simulink model "bh_source_WKSPACE"  (R2018a)
settings: Solver=ode4  StartTime=0.0  StopTime=80  FixedStep=0.001  RelTol=1e-5
settings Model: Creator=bhorton  LastModifiedBy=bhorton
settings SolverCC: ZeroCrossAlgorithm=Adaptive
settings OptimizationCC: LifeSpan=inf
settings DebuggingCC: SFUnexpectedBacktrackingDiag=warning  SFNoUnconditionalDefaultTransitionDiag=warning  SFExecutionAtInitializationDiag=none
settings CodeAppCC: StateflowObjectComments=on
settings GRTTargetCC: TargetLangStandard=C89/C90 (ANSI)
settings ConfigComp: CovMetricSettings=dw  CovHtmlReporting=on  CovSaveCumulativeToWorkspaceVar=on  CovSaveSingleToWorkspaceVar=on  CovExternalEMLEnable=off
settings SimscapeCC: SimscapeNormalizeSystem=off  SimscapeLogType=all  SimscapeLogDataHistory=10000  SelectedTab=Simscape Multibody
settings ExplorerConfigSet: InternalSimMechanicsExplorerSettings="<ExplorerConfiguration><canonicalview>default</canonicalview><AnimationSetting><BasePlaybackSpeed>1.0</BasePlaybackSpeed><PlaybackSpeedFactor>1.0</PlaybackSpeedFactor></AnimationSetting><TilePanel><TileInfo><Tiles Columns=\"2\" Count=\"4\" Rows=\"2\"><Column Left=\"2\" Weight=\"0.4992\"/><Column Left=\"655\" Weight=\"0.5008\"/><Column Left=\"1310\"/><Row Top=\"2\" Weight=\"0.4984\"/><Row Top=\"475\" Weight=\"0.5016\"/><Row Top=\"950\"/><Tile Height=\"1\" Width=\"1\" X=\"0\" Y=\"0\"/><Tile Height=\"1\" Width=\"1\" X=\"0\" Y=\"1\"/><Tile Height=\"1\" Width=\"1\" X=\"1\" Y=\"0\"/><Tile Height=\"1\" Width=\"1\" X=\"1\" Y=\"1\"/></Tiles></TileInfo><SceneInfo><SceneViewer><BGColor><R>0.60000002384185791</R><G>0.60000002384185791</G><B>0.60000002384185791</B></BGColor><Camera><DoPerspective>off</DoPerspective><Position><X>0.57010570867346566</X><Y>-0.81939487187068383</Y><Z>-0.041325690013103822</Z></Position><Center><X>0.57010570867346566</X><Y>0.37243777720020188</Y><Z>-0.041325690013103822</Z></Center><Up><X>0</X><Y>-0</Y><Z>1</Z></Up><ViewLimDist>1</ViewLimDist><YLim>0.58387397231837834</YLim><XLim>0.8103768064074045</XLim></Camera></SceneViewer><SceneViewer><BGColor><R>0.60000002384185791</R><G>0.60000002384185791</G><B>0.60000002384185791</B></BGColor><Camera><DoPerspective>off</DoPerspective><Position><X>0.51388092361444482</X><Y>0.52196280048326149</Y><Z>0.82022286793681332</Z></Position><Center><X>0.51388092361444482</X><Y>0.52196280048326149</Y><Z>-0.17977713206318668</Z></Center><Up><X>0</X><Y>1</Y><Z>-0</Z></Up><ViewLimDist>1</ViewLimDist><YLim>0.97737746692739225</YLim><XLim>1.3507104907751943</XLim></Camera></SceneViewer><SceneViewer><BGColor><R>0.60000002384185791</R><G>0.60000002384185791</G><B>0.60000002384185791</B></BGColor><Camera><DoPerspective>off</DoPerspective><Position><X>1.5094114010486579</X><Y>0.67796186035410533</Y><Z>-0.0082694811079057073</Z></Position><Center><X>0.47943838776152692</X><Y>0.67796186035410533</Y><Z>-0.0082694811079057073</Z></Center><Up><X>-0</X><Y>0</Y><Z>1</Z></Up><ViewLimDist>1</ViewLimDist><YLim>0.68608550995197048</YLim><XLim>0.95519663670037269</XLim></Camera></SceneViewer><SceneViewer><BGColor><R>0.60000002384185791</R><G>0.60000002384185791</G><B>0.60000002384185791</B></BGColor><Camera><DoPerspective>off</DoPerspective><Position><X>1.2860411296222924</X><Y>0.12259966358168611</Y><Z>0.94383913066063729</Z></Position><Center><X>0.57516484098717713</X><Y>0.83347595221680226</Y><Z>0.23296284202552392</Z></Center><Up><X>-0.40824829046386307</X><Y>0.40824829046386307</Y><Z>0.81649658092772615</Z></Up><ViewLimDist>1</ViewLimDist><YLim>0.94664886749230226</YLim><XLim>1.3123072283262387</XLim></Camera></SceneViewer></SceneInfo></TilePanel><MechEditorPanel><Cameras/><GfxPanelCameraMap/><VideoCreator><PlaybackSpeedRatio>1.0</PlaybackSpeedRatio><FrameRate>30</FrameRate><VideoFormat>Motion JPEG AVI</VideoFormat><FrameSize>auto</FrameSize></VideoCreator></MechEditorPanel></ExplorerConfiguration>"

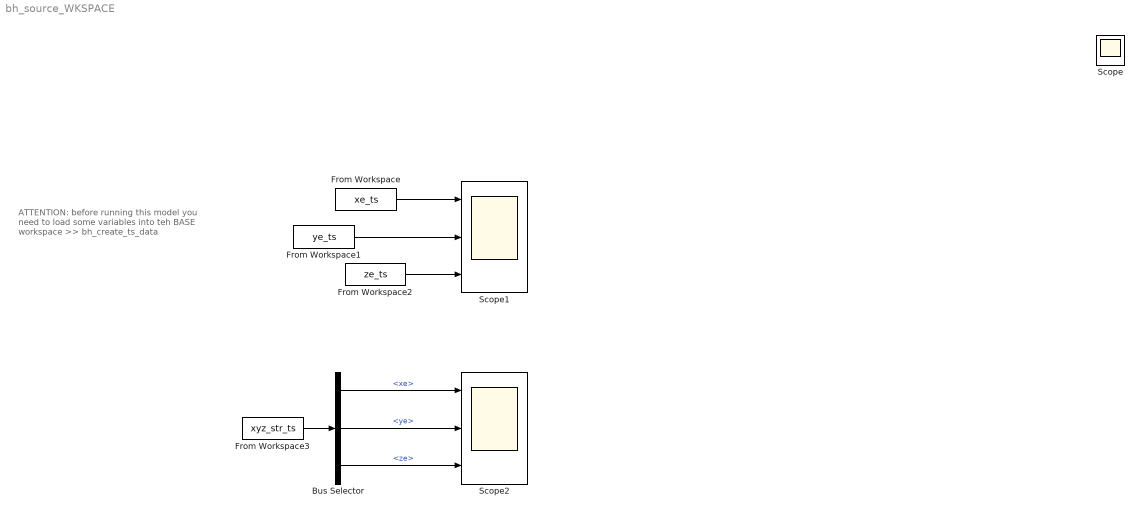
== system bh_source_WKSPACE ==
  note: ATTENTION:
      | before running this model you need to load
      | some variables into teh BASE workspace
      |
      | >>  bh_create_ts_data
  Bus Selector : BusSelector  OutputSignals=xe,ye,ze
  From Workspace : FromWorkspace  VariableName=xe_ts  SampleTime=0  OutputAfterFinalValue=Holding final value
  From Workspace1 : FromWorkspace  VariableName=ye_ts  SampleTime=0  OutputAfterFinalValue=Holding final value
  From Workspace2 : FromWorkspace  VariableName=ze_ts  SampleTime=0  OutputAfterFinalValue=Holding final value
  From Workspace3 : FromWorkspace  VariableName=xyz_str_ts  OutDataTypeStr=Bus: MY_XYZ_BUS_DEF  SampleTime=0  OutputAfterFinalValue=Holding final value
  Scope1 : Scope  NumInputPorts=3
  Scope2 : Scope  NumInputPorts=3
  Scope : Scope
  wires:
  From Workspace1/1 -> Scope1/2
  From Workspace2/1 -> Scope1/3
  From Workspace/1 -> Scope1/1
  From Workspace3/1 -> Bus Selector/1
  Bus Selector/2 -> Scope2/2  "<ye>"
  Bus Selector/1 -> Scope2/1  "<xe>"
  Bus Selector/3 -> Scope2/3  "<ze>"
